simulink model "processor_with_peripherals"  (R2025a)
settings: Solver=FixedStepDiscrete  StartTime=0.0  StopTime=inf  RelTol=1e-3
libraries: simulink x6
(part 1 of 5)
settings Model: Creator=Ananthan  LastModifiedBy=Ananthan

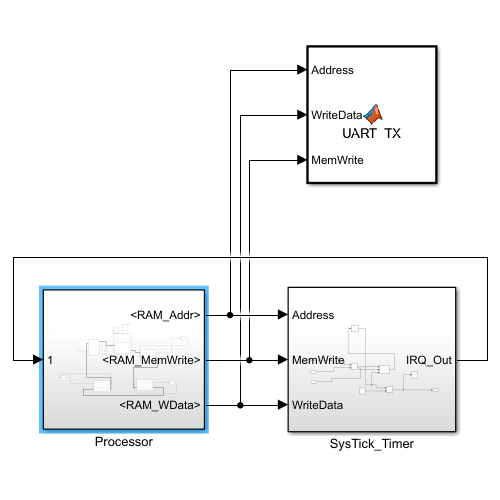
[thumbnail: Simulink's stored preview of the top-level diagram]
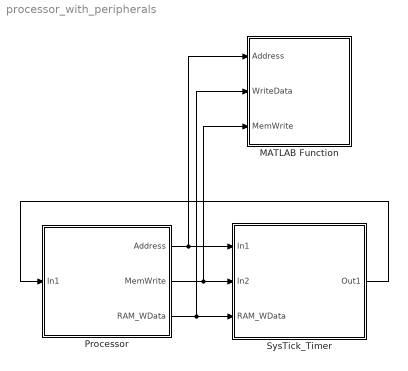
== system processor_with_peripherals ==
  MATLAB Function : MATLAB Function  TreatAsAtomicUnit=on
  Processor : Subsystem
  SysTick_Timer : Subsystem
  wires:
  Processor/1(Address) -> MATLAB Function/1(Address), SysTick_Timer/1(In1)
  Processor/2(MemWrite) -> MATLAB Function/3(MemWrite), SysTick_Timer/2(In2)
  Processor/3(RAM_WData) -> MATLAB Function/2(WriteData), SysTick_Timer/3(RAM_WData)
  SysTick_Timer/1(Out1) -> Processor/1(In1)
